simulink library "Disturbances"  (R2015a)
settings: Solver=ode45  StartTime=0.0  StopTime=10.0  RelTol=1e-3
undefined symbols (not defined in the file or in its folder): light_speed, sc_mass, slcm, solar_const
undefined symbols (not defined in the file): area, Constant, rad_press_coef, Sim
libraries: lib_gravity x3
settings Model: Creator=bbrito  LastModifiedBy=bbrito

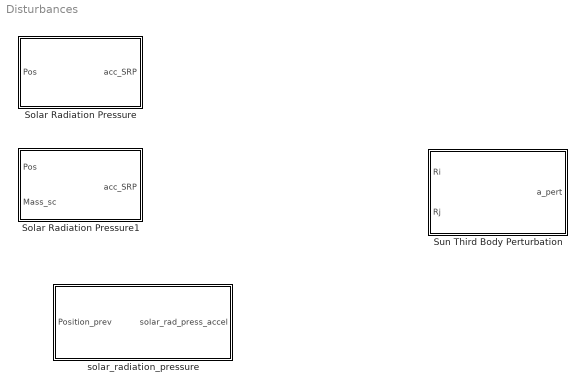
== system Disturbances ==
  Solar Radiation Pressure : Subsystem  TreatAsAtomicUnit=on  mask{A_sc=1, P0=0, M_sc=1}
      mask prompts: A_sc "Spacecraft Normal Area"; P0 "Solar Constant"; M_sc "Spacecraft Mass"
  Solar Radiation Pressure1 : Subsystem  AncestorBlock=Disturbances/Solar Radiation Pressure  TreatAsAtomicUnit=on  mask{A_sc=1, P0=0}
      mask prompts: A_sc "Spacecraft Normal Area"; P0 "Solar Constant"
  Sun Third Body Perturbation : Subsystem  TreatAsAtomicUnit=on  mask{g=Constant.SunGravity}
      mask prompts: g "Gravitational constant"
      mask help:
      | ESA-ESTEC
      | ---------------------------------------------------------------------------
      | Version:0.0          Date:8/10/20015          Author: #BB
      | Matlab version: 2015a          Project: AIM          Division: TEC-ECN
      | ---------------------------------------------------------------------------
      | This block models the shperical central body gravitation perturbation acceleration.
      |
      | The input is the perturbing body vector position Rj in cartesian coordinates.
      |
      | Ri is the point mass position vector in cartesian coordinates that is being perturbed.
  solar_radiation_pressure : Subsystem  mask(Copyright GMV, S.A. 2006.){solar_const=solar_const, astr_unit=astr_unit, cross_area=area, solar_rad_press_coef=rad_press_coef, light_speed=light_speed, sc_mass=sc_mass, timestep=Sim.Ts}
      mask prompts: solar_const "Solar constant (1,1) [W/m^2]"; astr_unit "Astronomical unit (1,1) [m]"; cross_area "Spacecraft cross area (1,1) [m^2]"; solar_rad_press_coef "Solar radiation pressure coeficient (1,1) [adimensional]"; light_speed "Speed of light (1,1) [m/s]"; sc_mass "Spacecraft mass (1,1) [kg]"; timestep "Step size (1,1) [s]"
      mask help:
      | V1.0 / MMGO.
      | This block models the solar radiation pressure acceleration.

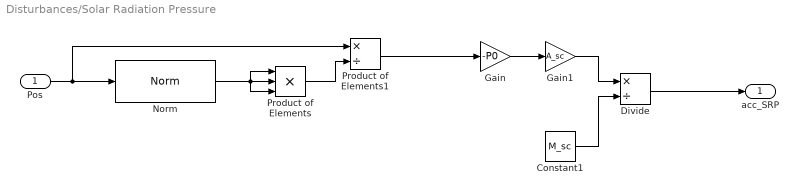
== system Disturbances/Solar Radiation Pressure ==
  Pos : Inport
  Constant1 : Constant  Value=M_sc
  Divide : Product  Inputs=*/
  Gain : Gain  Gain=-P0
  Gain1 : Gain  Gain=A_sc
  Norm : lib_gravity/Spherical Gravity Acceleration/Norm
  Product of Elements : Product  Inputs=***
  Product of Elements1 : Product  Inputs=*/
  acc_SRP : Outport
  wires:
  Gain/1 -> Gain1/1
  Gain1/1 -> Divide/1
  Constant1/1 -> Divide/2
  Norm/1 -> Product of Elements/3, Product of Elements/1, Product of Elements/2
  Product of Elements/1 -> Product of Elements1/2
  Pos/1 -> Product of Elements1/1, Norm/1
  Product of Elements1/1 -> Gain/1
  Divide/1 -> acc_SRP/1

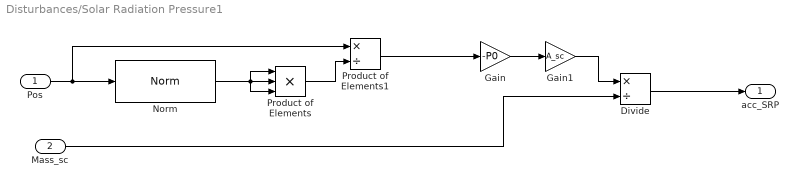
== system Disturbances/Solar Radiation Pressure1 ==
  Pos : Inport
  Mass_sc : Inport  Port=2
  Divide : Product  Inputs=*/
  Gain : Gain  Gain=-P0
  Gain1 : Gain  Gain=A_sc
  Norm : lib_gravity/Spherical Gravity Acceleration/Norm
  Product of Elements : Product  Inputs=***
  Product of Elements1 : Product  Inputs=*/
  acc_SRP : Outport
  wires:
  Gain/1 -> Gain1/1
  Gain1/1 -> Divide/1
  Norm/1 -> Product of Elements/3, Product of Elements/1, Product of Elements/2
  Product of Elements/1 -> Product of Elements1/2
  Pos/1 -> Product of Elements1/1, Norm/1
  Product of Elements1/1 -> Gain/1
  Divide/1 -> acc_SRP/1
  Mass_sc/1 -> Divide/2

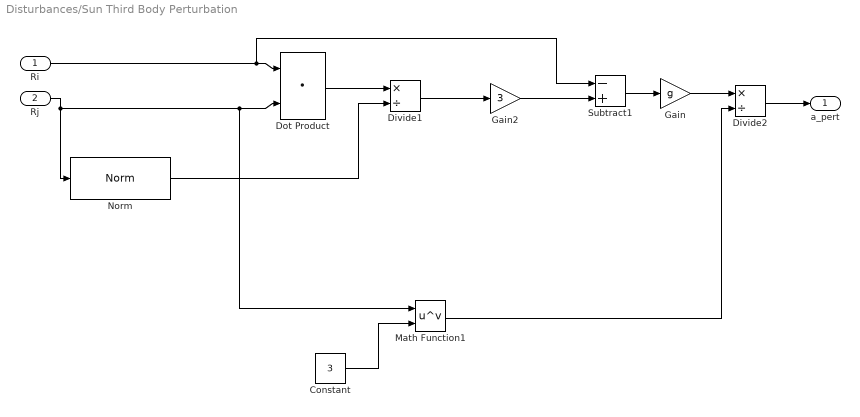
== system Disturbances/Sun Third Body Perturbation ==
  Ri : Inport
  Rj : Inport  Port=2
  Constant : Constant  Value=3
  Divide1 : Product  Inputs=*/
  Divide2 : Product  Inputs=*/
  Dot Product : DotProduct  InputSameDT=on  OutDataTypeStr=Inherit: Inherit via internal rule
  Gain : Gain  Gain=g
  Gain2 : Gain  Gain=3
  Math Function1 : Math  Operator=pow  SaturateOnIntegerOverflow=on
  Norm : lib_gravity/Spherical Gravity Acceleration/Norm
  Subtract1 : Sum  Inputs=-+
  a_pert : Outport
  wires:
  Ri/1 -> Subtract1/1, Dot Product/1
  Dot Product/1 -> Divide1/1
  Gain/1 -> Divide2/1
  Rj/1 -> Math Function1/1, Dot Product/2, Norm/1
  Norm/1 -> Divide1/2
  Divide1/1 -> Gain2/1
  Gain2/1 -> Subtract1/2
  Subtract1/1 -> Gain/1
  Constant/1 -> Math Function1/2
  Math Function1/1 -> Divide2/2
  Divide2/1 -> a_pert/1

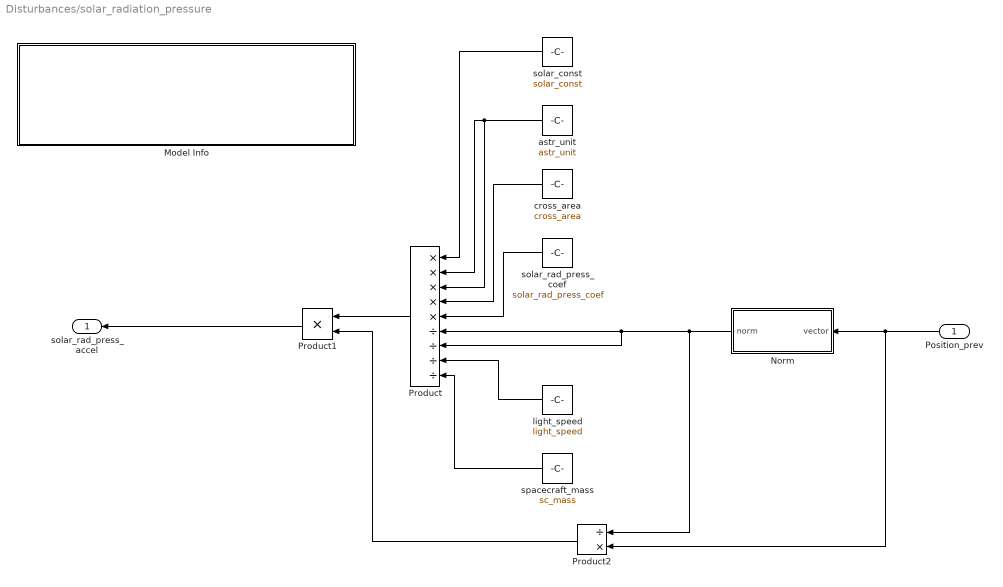
== system Disturbances/solar_radiation_pressure ==
  Position_prev : Inport
  Model Info : Subsystem  LoadFcn=slcm LoadBlock;  InitFcn=slcm('UpdateAllCMBlocksInThisModelInit')  mask(CMBlock){InitialSaveTempField=, InitialBlockCM=, BlockCM=, Frame=on, SaveTempField=, DisplayStringWithTags=|, MaskDisplayString=Copyright GMV, S.A. 2006.\n---------------------------------------------------------------------------\nVersion:1.0          Date:26/7/2006          Author: MMGO\nSimulink Ver.:6.3          Project:CHILON          Division: MAAS\n---------------------------------------------------------------------------\nThis block models the solar radiation pressure acceleration., HorizontalTextAlignment=Center, LeftAlignmentValue=0.5, SourceBlockDiagram=Disturbances, TagMaxNumber=20, CMTag1=, CMTag2=, CMTag3=, CMTag4=, CMTag5=, CMTag6=, CMTag7=, CMTag8=, CMTag9=, CMTag10=, CMTag11=, CMTag12=, CMTag13=, CMTag14=, CMTag15=, CMTag16=, CMTag17=, CMTag18=, CMTag19=, CMTag20=}
      mask DisplayStringWithTags=|
      | Copyright GMV, S.A. 2006.
      | ---------------------------------------------------------------------------
      | Version:1.0          Date:26/7/2006          Author: MMGO
      | Simulink Ver.:6.3          Project:CHILON          Division: MAAS
      | ---------------------------------------------------------------------------
      | This block models the solar radiation pressure acceleration.
      mask prompts: InitialSaveTempField "Simulink:masks:InitialSaveTempField_MP"; InitialBlockCM "Simulink:masks:InitialBlockCM_MP"; BlockCM "Simulink:masks:BlockCM_MP"; Frame "Simulink:masks:Frame_MP"; SaveTempField "Simulink:masks:SaveTempField_MP"; DisplayStringWithTags "Simulink:masks:DisplayStringWithTags_MP"; MaskDisplayString "Simulink:masks:MaskDisplayString_MP"; HorizontalTextAlignment "Simulink:masks:HorizontalTextAlignment_MP"; LeftAlignmentValue "Simulink:masks:LeftAlignmentValue_MP"; SourceBlockDiagram "Simulink:masks:SourceBlockDiagram_MP"; TagMaxNumber "Simulink:masks:TagMaxNumber_MP"; CMTag1 "Simulink:masks:CMTag1_MP"; CMTag2 "Simulink:masks:CMTag2_MP"; CMTag3 "Simulink:masks:CMTag3_MP"; CMTag4 "Simulink:masks:CMTag4_MP"; CMTag5 "Simulink:masks:CMTag5_MP"; CMTag6 "Simulink:masks:CMTag6_MP"; CMTag7 "Simulink:masks:CMTag7_MP"; CMTag8 "Simulink:masks:CMTag8_MP"; CMTag9 "Simulink:masks:CMTag9_MP"; CMTag10 "Simulink:masks:CMTag10_MP"; CMTag11 "Simulink:masks:CMTag11_MP"; CMTag12 "Simulink:masks:CMTag12_MP"; CMTag13 "Simulink:masks:CMTag13_MP"; CMTag14 "Simulink:masks:CMTag14_MP"; CMTag15 "Simulink:masks:CMTag15_MP"; CMTag16 "Simulink:masks:CMTag16_MP"; CMTag17 "Simulink:masks:CMTag17_MP"; CMTag18 "Simulink:masks:CMTag18_MP"; CMTag19 "Simulink:masks:CMTag19_MP"; CMTag20 "Simulink:masks:CMTag20_MP"
      mask help: Simulink:masks:CMBlock_MD
      settings: CopyFcn=slcm CopyBlock;  DeleteFcn=slcm Cancel;  PostSaveFcn=slcm('UpdateAllCMBlocksInThisModel')  NameChangeFcn=slcm Rename;  OpenFcn=slcm
      mask Display: text(str2num(LeftAlignmentValue), 0.5, MaskDisplayString, 'HorizontalAlignment', HorizontalTextAlignment)
  Norm : Subsystem
  Product : Product  Inputs=*****////  RndMeth=Zero
  Product1 : Product  RndMeth=Zero
  Product2 : Product  Inputs=/*  RndMeth=Zero
  astr_unit : Constant  Value=astr_unit
  cross_area : Constant  Value=cross_area
  light_speed : Constant  Value=light_speed
  solar_const : Constant  Value=solar_const
  solar_rad_press_coef : Constant  Value=solar_rad_press_coef
  spacecraft_mass : Constant  Value=sc_mass
  solar_rad_press_accel : Outport
  wires:
  Product2/1 -> Product1/2
  Product1/1 -> solar_rad_press_accel/1
  Product/1 -> Product1/1
  Position_prev/1 -> Norm/1(vector), Product2/2
  spacecraft_mass/1 -> Product/9
  light_speed/1 -> Product/8
  Norm/1(norm) -> Product2/1, Product/7, Product/6
  solar_const/1 -> Product/1
  astr_unit/1 -> Product/2, Product/3
  cross_area/1 -> Product/4
  solar_rad_press_coef/1 -> Product/5

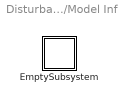
== system Disturbances/solar_radiation_pressure/Model Info ==
  EmptySubsystem : Subsystem

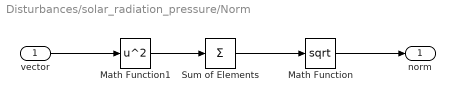
== system Disturbances/solar_radiation_pressure/Norm ==
  vector : Inport
  Math Function : Math  Operator=sqrt  SaturateOnIntegerOverflow=on
  Math Function1 : Math  Operator=square  SaturateOnIntegerOverflow=on
  Sum of Elements : Sum  Inputs=+
  norm : Outport
  wires:
  Sum of Elements/1 -> Math Function/1
  Math Function1/1 -> Sum of Elements/1
  vector/1 -> Math Function1/1
  Math Function/1 -> norm/1

== system Disturbances/solar_radiation_pressure/Model Info/EmptySubsystem ==
